simulink model "VSC_slk"  (R2023b)
settings: Solver=FixedStepAuto  StartTime=0.0  StopTime=Tend_slk  FixedStep=0.01  RelTol=1e-3
values from neighbouring files (symbols this model uses):
  A = [0 1 ... (first row only)    [main_VSC.m]
  alpha = beta*A    [main_VSC.m]
  B = [0 ... (first row only)    [main_VSC.m]
  beta = [0.5 1]    [main_VSC.m]
  gamma = 0.5    [main_VSC.m]
  q = 7.5e-3*y_des/t_reach+W    (= 0.2075)    [main_VSC.m]
  r = 1    [main_VSC.m]
  Ts_slk = 0.01    [main_VSC.m]
  y_des = 0.5/0.5    (= 1)    [main_VSC.m]
settings Model: Creator=asus  LastModifiedBy=asus

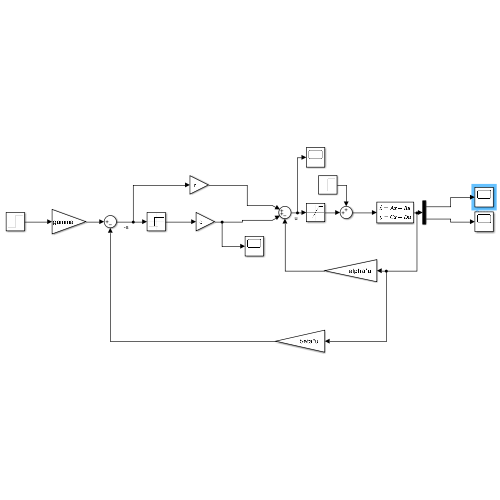
[thumbnail: Simulink's stored preview of the top-level diagram]
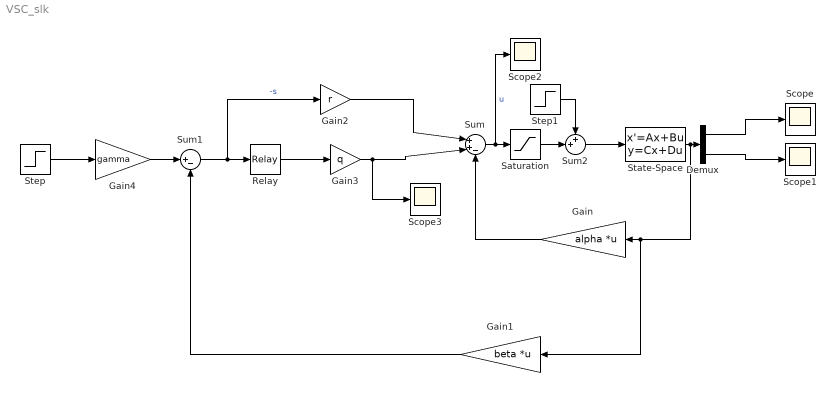
== system VSC_slk ==
  Demux : Demux  Outputs=2
  Gain : Gain  Gain=alpha  Multiplication=Matrix(K*u)
  Gain1 : Gain  Gain=beta  Multiplication=Matrix(K*u)
  Gain2 : Gain  Gain=r
  Gain3 : Gain  Gain=q
  Gain4 : Gain  Gain=gamma
  Relay : Relay  OnSwitchValue=0.1  OffSwitchValue=-0.1  OffOutputValue=-1
  Saturation : Saturate  UpperLimit=0.85  LowerLimit=-0.85
  Scope{,1..3} (4 alike) : Scope
  State-Space : StateSpace  A=A  B=B  C=eye(2)  D=[0;0]  InitialCondition=0  ParameterTunability=Unconstrained
  Step : Step  Time=0  After=y_des  SampleTime=Ts_slk
  Step1 : Step  Time=0  After=0.002*0  SampleTime=0
  Sum : Sum  Inputs=|++-
  Sum1 : Sum  Inputs=|+-
  Sum2 : Sum  Inputs=++|
  wires:
  Gain/1 -> Sum/3
  Sum/1 -> Scope2/1, Saturation/1  "u"
  Relay/1 -> Gain3/1
  Sum1/1 -> Relay/1, Gain2/1  "-s"
  Step/1 -> Gain4/1
  Gain4/1 -> Sum1/1
  Gain1/1 -> Sum1/2
  Gain2/1 -> Sum/1
  State-Space/1 -> Demux/1, Gain1/1, Gain/1
  Demux/1 -> Scope/1
  Demux/2 -> Scope1/1
  Saturation/1 -> Sum2/2
  Sum2/1 -> State-Space/1
  Step1/1 -> Sum2/1
  Gain3/1 -> Scope3/1, Sum/2
